simulink subsystem "loggingsub"  (R2020b)
settings: Solver=VariableStepAuto  StartTime=0.0  StopTime=10.0  RelTol=1e-3
settings Model: Creator=MSI PC  LastModifiedBy=MSI PC

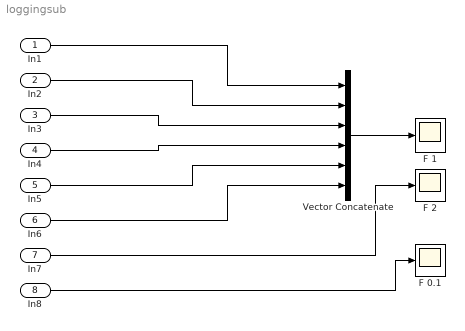
== system loggingsub ==
  In1 : Inport
  In2 : Inport  Port=2
  In3 : Inport  Port=3
  In4 : Inport  Port=4
  In5 : Inport  Port=5
  In6 : Inport  Port=6
  In7 : Inport  Port=7
  In8 : Inport  Port=8
  F 0.1 : Scope
  F 1 : Scope
  F 2 : Scope
  Vector Concatenate : Concatenate  NumInputs=6
  wires:
  Vector Concatenate/1 -> F 1/1
  In5/1 -> Vector Concatenate/5
  In2/1 -> Vector Concatenate/2
  In8/1 -> F 0.1/1
  In4/1 -> Vector Concatenate/4
  In3/1 -> Vector Concatenate/3
  In6/1 -> Vector Concatenate/6
  In1/1 -> Vector Concatenate/1
  In7/1 -> F 2/1
